simulink model "PID_fin"  (R2023b)
settings: Solver=VariableStepAuto  StartTime=0.0  StopTime=20  RelTol=1e-3
values from neighbouring files (symbols this model uses):
  A = double(A)    [Rotational_inverted_pendulum.m]
  B = double(B)    [Rotational_inverted_pendulum.m]
  C = [1 0 0 0 ... (first row only)    [Rotational_inverted_pendulum.m]
  D = [0 ... (first row only)    [Rotational_inverted_pendulum.m]
  den_phi = cell2mat(G_t2p_uns.Denominator)    [Rotational_inverted_pendulum.m]
  den_theta = cell2mat(G_ol_uns.Denominator(1,1))    [Rotational_inverted_pendulum.m]
  Kd_phi = 60    [Rotational_inverted_pendulum.m]
  Kd_phi_v2 = 0    [Rotational_inverted_pendulum.m]
  Kd_theta = 2    [Rotational_inverted_pendulum.m]
  Kd_theta_v2 = 0.25    [Rotational_inverted_pendulum.m]
  Ki_phi = 50    [Rotational_inverted_pendulum.m]
  Ki_phi_v2 = 7    [Rotational_inverted_pendulum.m]
  Ki_theta = 0    [Rotational_inverted_pendulum.m]
  Ki_theta_v2 = 0    [Rotational_inverted_pendulum.m]
  Kp_phi = 90    [Rotational_inverted_pendulum.m]
  Kp_phi_v2 = 0    [Rotational_inverted_pendulum.m]
  Kp_theta = 5    [Rotational_inverted_pendulum.m]
  Kp_theta_v2 = 0.9    [Rotational_inverted_pendulum.m]
  num_phi = cell2mat(G_t2p_uns.Numerator)    [Rotational_inverted_pendulum.m]
  num_theta = cell2mat(G_ol_uns.Numerator(1,1))    [Rotational_inverted_pendulum.m]
  Va_bar = 0    [Rotational_inverted_pendulum.m]
  x1_bar = double(sol.x1)    [Rotational_inverted_pendulum.m]
  x3_bar = 0    [Rotational_inverted_pendulum.m]
libraries: simulink_extras x5, slpidlib x4
settings Model: Creator=Mark  LastModifiedBy=Mark

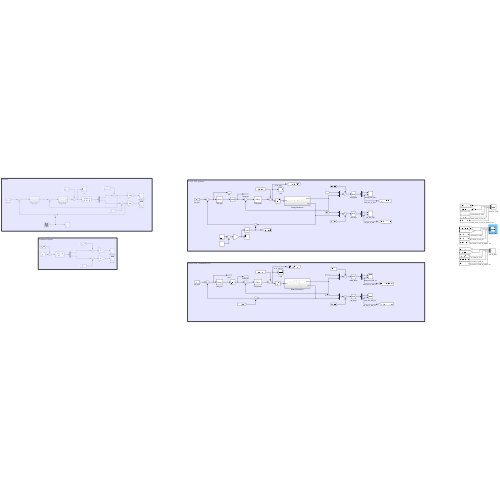
[thumbnail: Simulink's stored preview of the top-level diagram]
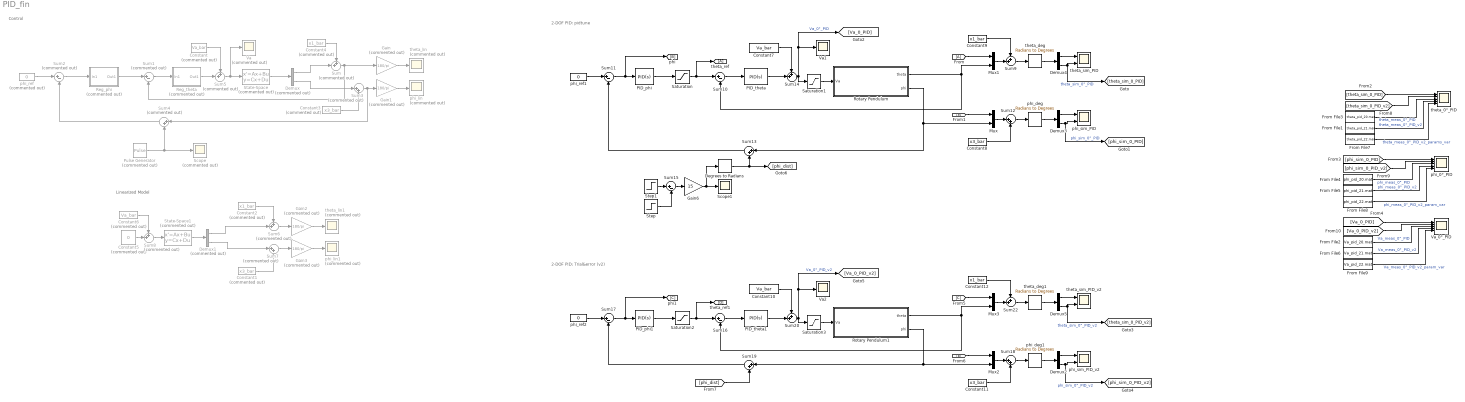
== system PID_fin ==
  note: Control
  note: Linearized Model
  note: 2-DOF PID: pidtune
  note: 2-DOF PID: Trial&error (v2)
  Constant : Constant  Commented=on  Value=Va_bar
  Constant1 : Constant  Commented=on  Value=x3_bar
  Constant10 : Constant  Value=Va_bar
  Constant11 : Constant  Value=x3_bar
  Constant12 : Constant  Value=x1_bar
  Constant2 : Constant  Commented=on  Value=x1_bar
  Constant3 : Constant  Commented=on  Value=x3_bar
  Constant4 : Constant  Commented=on  Value=x1_bar
  Constant5 : Constant  Commented=on  Value=0
  Constant6 : Constant  Commented=on  Value=Va_bar
  Constant7 : Constant  Value=Va_bar
  Constant8 : Constant  Value=x3_bar
  Constant9 : Constant  Value=x1_bar
  Degrees to Radians : simulink_extras/Transformations/Degrees to Radians
  Demux : Demux  Commented=on  Outputs=2
  Demux1 : Demux  Commented=on  Outputs=2
  Demux{2..5} (4 alike) : Demux  Outputs=2
  From : From
  From File1 : FromFile  FileName=theta_pid_21.mat  SampleTime=0
  From File2 : FromFile  FileName=Va_pid_20.mat  SampleTime=0
  From File3 : FromFile  FileName=theta_pid_20.mat  SampleTime=0
  From File4 : FromFile  FileName=phi_pid_20.mat  SampleTime=0
  From File5 : FromFile  FileName=phi_pid_21.mat  SampleTime=0
  From File6 : FromFile  FileName=Va_pid_21.mat  SampleTime=0
  From File7 : FromFile  FileName=theta_pid_22.mat  SampleTime=0
  From File8 : FromFile  FileName=phi_pid_22.mat  SampleTime=0
  From File9 : FromFile  FileName=Va_pid_22.mat  SampleTime=0
  Gain{,1..3} (4 alike) : Gain  Commented=on  Gain=180/pi
  Gain6 : Gain  Gain=15
  Mux{,1..3} (4 alike) : Mux  Inputs=2
  PID_phi : slpidlib/PID Controller  Controller=PID  Form=Parallel  TimeDomain=Continuous-time  UseExternalTs=off  SampleTime=-1  IntegratorMethod=Forward Euler  FilterMethod=Forward Euler  ControllerParametersSource=internal  P=Kp_phi  I=Ki_phi  UseKiTs=off  D=Kd_phi  N=100  UseFilter=on  TunerSelectOption=Transfer Function Based (PID Tuner App)  InitialConditionSource=internal  InitialConditionForIntegrator=0  InitialConditionForFilter=0  DifferentiatorICPrevScaledInput=0  ExternalReset=none  TrackingMode=off  Kt=1  LimitOutput=off  SatLimitsSource=internal  UpperSaturationLimit=90  LowerSaturationLimit=-90  LinearizeAsGain=on  AntiWindupMode=none  Kb=1  LimitIntegrator=off  UpperIntegratorSaturationLimit=inf  LowerIntegratorSaturationLimit=-inf  POutMin=[]  POutMax=[]  IOutMin=[]  IOutMax=[]  DOutMin=[]  DOutMax=[]  NOutMin=[]  NOutMax=[]  SumOutMin=[]  SumOutMax=[]  SaturationOutMin=[]  SaturationOutMax=[]  PParamMin=[]  PParamMax=[]  IParamMin=[]  IParamMax=[]  DParamMin=[]  DParamMax=[]  NParamMin=[]  NParamMax=[]  KbParamMin=[]  KbParamMax=[]  KtParamMin=[]  KtParamMax=[]  KbOutMin=[]  KbOutMax=[]  KtOutMin=[]  KtOutMax=[]  IntegratorOutMin=[]  IntegratorOutMax=[]  FilterOutMin=[]  FilterOutMax=[]  SumI1OutMin=[]  SumI1OutMax=[]  SumI2OutMin=[]  SumI2OutMax=[]  SumI3OutMin=[]  SumI3OutMax=[]  SumI4OutMin=[]  SumI4OutMax=[]  SumDOutMin=[]  SumDOutMax=[]  DifferentiatorOutMin=[]  DifferentiatorOutMax=[]  FilterDiffOutCoefMin=[]  FilterDiffOutCoefMax=[]  ReciprocalOutMin=[]  ReciprocalOutMax=[]  SumDenOutMin=[]  SumDenOutMax=[]  SumNumOutMin=[]  SumNumOutMax=[]  DivideOutMin=[]  DivideOutMax=[]  UdiffTsProdOutMin=[]  UdiffTsProdOutMax=[]  NTsProdOutMin=[]  NTsProdOutMax=[]  UintegralTsProdOutMin=[]  UintegralTsProdOutMax=[]  UngainTsProdOutMin=[]  UngainTsProdOutMax=[]  ClampingZeroOutDataTypeStr=Inherit: Inherit via back propagation  ClampingZeroOutMin=[]  ClampingZeroOutMax=[]  FilterDenConstantOutDataTypeStr=Inherit: Inherit via back propagation  FilterDenConstantOutMin=[]  FilterDenConstantOutMax=[]  PCopyOutDataTypeStr=Inherit: Inherit via back propagation  PCopyOutMin=[]  PCopyOutMax=[]  NCopyOutDataTypeStr=Inherit: Inherit via back propagation  NCopyOutMin=[]  NCopyOutMax=[]  IntegratorContinuousStateAttributes=''  IntegratorStateMustResolveToSignalObject=off  IntegratorRTWStateStorageClass=Auto  FilterContinuousStateAttributes=''  FilterStateMustResolveToSignalObject=off  FilterRTWStateStorageClass=Auto  ParallelPVariant=InternalParameters  IdealPVariant=Disabled  IVariant=InternalParameters  DVariant=InternalParameters  IntegratorVariant=Continuous  SatVariant=Disabled  AWVariant=Passthrough  PCopyVariant=Disabled  TRVariant=Disabled  FdbkBlocksVariant=Forward  IdealPFdbkVariant=Disabled  SatFdbkVariant=Disabled  DerivativeFilterVariant=ContFilter  NVariant=InternalParameters  NCopyVariant=Disabled  FilterICVariant=InternalICsFilter  IntegratorICVariant=InternalICs  ExternalResetVariant=Disabled  TRSumVariant=Passthrough  SumFdbkVariant=Disabled  SumVariant=Sum_PID  TsampFilterVariant=InternalTs  TsampNgainVariant=Passthrough  TsampIntegralVariant=Disabled_SignalSpec  ExternalSaturationOutDataTypeStr=Inherit: Same as second input
  PID_phi1 : slpidlib/PID Controller  Controller=PID  Form=Parallel  TimeDomain=Continuous-time  UseExternalTs=off  SampleTime=-1  IntegratorMethod=Forward Euler  FilterMethod=Forward Euler  ControllerParametersSource=internal  P=Kp_phi_v2  I=Ki_phi_v2  UseKiTs=off  D=Kd_phi_v2  N=100  UseFilter=on  TunerSelectOption=Transfer Function Based (PID Tuner App)  InitialConditionSource=internal  InitialConditionForIntegrator=0  InitialConditionForFilter=0  DifferentiatorICPrevScaledInput=0  ExternalReset=none  TrackingMode=off  Kt=1  LimitOutput=off  SatLimitsSource=internal  UpperSaturationLimit=90  LowerSaturationLimit=-90  LinearizeAsGain=on  AntiWindupMode=none  Kb=1  LimitIntegrator=off  UpperIntegratorSaturationLimit=inf  LowerIntegratorSaturationLimit=-inf  POutMin=[]  POutMax=[]  IOutMin=[]  IOutMax=[]  DOutMin=[]  DOutMax=[]  NOutMin=[]  NOutMax=[]  SumOutMin=[]  SumOutMax=[]  SaturationOutMin=[]  SaturationOutMax=[]  PParamMin=[]  PParamMax=[]  IParamMin=[]  IParamMax=[]  DParamMin=[]  DParamMax=[]  NParamMin=[]  NParamMax=[]  KbParamMin=[]  KbParamMax=[]  KtParamMin=[]  KtParamMax=[]  KbOutMin=[]  KbOutMax=[]  KtOutMin=[]  KtOutMax=[]  IntegratorOutMin=[]  IntegratorOutMax=[]  FilterOutMin=[]  FilterOutMax=[]  SumI1OutMin=[]  SumI1OutMax=[]  SumI2OutMin=[]  SumI2OutMax=[]  SumI3OutMin=[]  SumI3OutMax=[]  SumI4OutMin=[]  SumI4OutMax=[]  SumDOutMin=[]  SumDOutMax=[]  DifferentiatorOutMin=[]  DifferentiatorOutMax=[]  FilterDiffOutCoefMin=[]  FilterDiffOutCoefMax=[]  ReciprocalOutMin=[]  ReciprocalOutMax=[]  SumDenOutMin=[]  SumDenOutMax=[]  SumNumOutMin=[]  SumNumOutMax=[]  DivideOutMin=[]  DivideOutMax=[]  UdiffTsProdOutMin=[]  UdiffTsProdOutMax=[]  NTsProdOutMin=[]  NTsProdOutMax=[]  UintegralTsProdOutMin=[]  UintegralTsProdOutMax=[]  UngainTsProdOutMin=[]  UngainTsProdOutMax=[]  ClampingZeroOutDataTypeStr=Inherit: Inherit via back propagation  ClampingZeroOutMin=[]  ClampingZeroOutMax=[]  FilterDenConstantOutDataTypeStr=Inherit: Inherit via back propagation  FilterDenConstantOutMin=[]  FilterDenConstantOutMax=[]  PCopyOutDataTypeStr=Inherit: Inherit via back propagation  PCopyOutMin=[]  PCopyOutMax=[]  NCopyOutDataTypeStr=Inherit: Inherit via back propagation  NCopyOutMin=[]  NCopyOutMax=[]  IntegratorContinuousStateAttributes=''  IntegratorStateMustResolveToSignalObject=off  IntegratorRTWStateStorageClass=Auto  FilterContinuousStateAttributes=''  FilterStateMustResolveToSignalObject=off  FilterRTWStateStorageClass=Auto  ParallelPVariant=InternalParameters  IdealPVariant=Disabled  IVariant=InternalParameters  DVariant=InternalParameters  IntegratorVariant=Continuous  SatVariant=Disabled  AWVariant=Passthrough  PCopyVariant=Disabled  TRVariant=Disabled  FdbkBlocksVariant=Forward  IdealPFdbkVariant=Disabled  SatFdbkVariant=Disabled  DerivativeFilterVariant=ContFilter  NVariant=InternalParameters  NCopyVariant=Disabled  FilterICVariant=InternalICsFilter  IntegratorICVariant=InternalICs  ExternalResetVariant=Disabled  TRSumVariant=Passthrough  SumFdbkVariant=Disabled  SumVariant=Sum_PID  TsampFilterVariant=InternalTs  TsampNgainVariant=Passthrough  TsampIntegralVariant=Disabled_SignalSpec  ExternalSaturationOutDataTypeStr=Inherit: Same as second input
  PID_theta : slpidlib/PID Controller  Controller=PID  Form=Parallel  TimeDomain=Continuous-time  UseExternalTs=off  SampleTime=-1  IntegratorMethod=Forward Euler  FilterMethod=Forward Euler  ControllerParametersSource=internal  P=Kp_theta  I=Ki_theta  UseKiTs=off  D=Kd_theta  N=100  UseFilter=on  TunerSelectOption=Frequency Response Based  InitialConditionSource=internal  InitialConditionForIntegrator=0  InitialConditionForFilter=0  DifferentiatorICPrevScaledInput=0  ExternalReset=none  TrackingMode=off  Kt=1  LimitOutput=off  SatLimitsSource=internal  UpperSaturationLimit=10  LowerSaturationLimit=-10  LinearizeAsGain=on  AntiWindupMode=back-calculation  Kb=Ki_theta/Kp_theta  LimitIntegrator=off  UpperIntegratorSaturationLimit=inf  LowerIntegratorSaturationLimit=-inf  POutMin=[]  POutMax=[]  IOutMin=[]  IOutMax=[]  DOutMin=[]  DOutMax=[]  NOutMin=[]  NOutMax=[]  SumOutMin=[]  SumOutMax=[]  SaturationOutMin=[]  SaturationOutMax=[]  PParamMin=[]  PParamMax=[]  IParamMin=[]  IParamMax=[]  DParamMin=[]  DParamMax=[]  NParamMin=[]  NParamMax=[]  KbParamMin=[]  KbParamMax=[]  KtParamMin=[]  KtParamMax=[]  KbOutMin=[]  KbOutMax=[]  KtOutMin=[]  KtOutMax=[]  IntegratorOutMin=[]  IntegratorOutMax=[]  FilterOutMin=[]  FilterOutMax=[]  SumI1OutMin=[]  SumI1OutMax=[]  SumI2OutMin=[]  SumI2OutMax=[]  SumI3OutMin=[]  SumI3OutMax=[]  SumI4OutMin=[]  SumI4OutMax=[]  SumDOutMin=[]  SumDOutMax=[]  DifferentiatorOutMin=[]  DifferentiatorOutMax=[]  FilterDiffOutCoefMin=[]  FilterDiffOutCoefMax=[]  ReciprocalOutMin=[]  ReciprocalOutMax=[]  SumDenOutMin=[]  SumDenOutMax=[]  SumNumOutMin=[]  SumNumOutMax=[]  DivideOutMin=[]  DivideOutMax=[]  UdiffTsProdOutMin=[]  UdiffTsProdOutMax=[]  NTsProdOutMin=[]  NTsProdOutMax=[]  UintegralTsProdOutMin=[]  UintegralTsProdOutMax=[]  UngainTsProdOutMin=[]  UngainTsProdOutMax=[]  ClampingZeroOutDataTypeStr=Inherit: Inherit via back propagation  ClampingZeroOutMin=[]  ClampingZeroOutMax=[]  FilterDenConstantOutDataTypeStr=Inherit: Inherit via back propagation  FilterDenConstantOutMin=[]  FilterDenConstantOutMax=[]  PCopyOutDataTypeStr=Inherit: Inherit via back propagation  PCopyOutMin=[]  PCopyOutMax=[]  NCopyOutDataTypeStr=Inherit: Inherit via back propagation  NCopyOutMin=[]  NCopyOutMax=[]  IntegratorContinuousStateAttributes=''  IntegratorStateMustResolveToSignalObject=off  IntegratorRTWStateStorageClass=Auto  FilterContinuousStateAttributes=''  FilterStateMustResolveToSignalObject=off  FilterRTWStateStorageClass=Auto  ParallelPVariant=InternalParameters  IdealPVariant=Disabled  IVariant=InternalParameters  DVariant=InternalParameters  IntegratorVariant=Continuous  SatVariant=Disabled  AWVariant=Passthrough  PCopyVariant=Disabled  TRVariant=Disabled  FdbkBlocksVariant=Forward  IdealPFdbkVariant=Disabled  SatFdbkVariant=Disabled  DerivativeFilterVariant=ContFilter  NVariant=InternalParameters  NCopyVariant=Disabled  FilterICVariant=InternalICsFilter  IntegratorICVariant=InternalICs  ExternalResetVariant=Disabled  TRSumVariant=Passthrough  SumFdbkVariant=Disabled  SumVariant=Sum_PID  TsampFilterVariant=InternalTs  TsampNgainVariant=Passthrough  TsampIntegralVariant=Disabled_SignalSpec  ExternalSaturationOutDataTypeStr=Inherit: Same as second input
  PID_theta1 : slpidlib/PID Controller  Controller=PID  Form=Parallel  TimeDomain=Continuous-time  UseExternalTs=off  SampleTime=-1  IntegratorMethod=Forward Euler  FilterMethod=Forward Euler  ControllerParametersSource=internal  P=Kp_theta_v2  I=Ki_theta_v2  UseKiTs=off  D=Kd_theta_v2  N=100  UseFilter=on  TunerSelectOption=Frequency Response Based  InitialConditionSource=internal  InitialConditionForIntegrator=0  InitialConditionForFilter=0  DifferentiatorICPrevScaledInput=0  ExternalReset=none  TrackingMode=off  Kt=1  LimitOutput=off  SatLimitsSource=internal  UpperSaturationLimit=10  LowerSaturationLimit=-10  LinearizeAsGain=on  AntiWindupMode=back-calculation  Kb=Ki_theta/Kp_theta  LimitIntegrator=off  UpperIntegratorSaturationLimit=inf  LowerIntegratorSaturationLimit=-inf  POutMin=[]  POutMax=[]  IOutMin=[]  IOutMax=[]  DOutMin=[]  DOutMax=[]  NOutMin=[]  NOutMax=[]  SumOutMin=[]  SumOutMax=[]  SaturationOutMin=[]  SaturationOutMax=[]  PParamMin=[]  PParamMax=[]  IParamMin=[]  IParamMax=[]  DParamMin=[]  DParamMax=[]  NParamMin=[]  NParamMax=[]  KbParamMin=[]  KbParamMax=[]  KtParamMin=[]  KtParamMax=[]  KbOutMin=[]  KbOutMax=[]  KtOutMin=[]  KtOutMax=[]  IntegratorOutMin=[]  IntegratorOutMax=[]  FilterOutMin=[]  FilterOutMax=[]  SumI1OutMin=[]  SumI1OutMax=[]  SumI2OutMin=[]  SumI2OutMax=[]  SumI3OutMin=[]  SumI3OutMax=[]  SumI4OutMin=[]  SumI4OutMax=[]  SumDOutMin=[]  SumDOutMax=[]  DifferentiatorOutMin=[]  DifferentiatorOutMax=[]  FilterDiffOutCoefMin=[]  FilterDiffOutCoefMax=[]  ReciprocalOutMin=[]  ReciprocalOutMax=[]  SumDenOutMin=[]  SumDenOutMax=[]  SumNumOutMin=[]  SumNumOutMax=[]  DivideOutMin=[]  DivideOutMax=[]  UdiffTsProdOutMin=[]  UdiffTsProdOutMax=[]  NTsProdOutMin=[]  NTsProdOutMax=[]  UintegralTsProdOutMin=[]  UintegralTsProdOutMax=[]  UngainTsProdOutMin=[]  UngainTsProdOutMax=[]  ClampingZeroOutDataTypeStr=Inherit: Inherit via back propagation  ClampingZeroOutMin=[]  ClampingZeroOutMax=[]  FilterDenConstantOutDataTypeStr=Inherit: Inherit via back propagation  FilterDenConstantOutMin=[]  FilterDenConstantOutMax=[]  PCopyOutDataTypeStr=Inherit: Inherit via back propagation  PCopyOutMin=[]  PCopyOutMax=[]  NCopyOutDataTypeStr=Inherit: Inherit via back propagation  NCopyOutMin=[]  NCopyOutMax=[]  IntegratorContinuousStateAttributes=''  IntegratorStateMustResolveToSignalObject=off  IntegratorRTWStateStorageClass=Auto  FilterContinuousStateAttributes=''  FilterStateMustResolveToSignalObject=off  FilterRTWStateStorageClass=Auto  ParallelPVariant=InternalParameters  IdealPVariant=Disabled  IVariant=InternalParameters  DVariant=InternalParameters  IntegratorVariant=Continuous  SatVariant=Disabled  AWVariant=Passthrough  PCopyVariant=Disabled  TRVariant=Disabled  FdbkBlocksVariant=Forward  IdealPFdbkVariant=Disabled  SatFdbkVariant=Disabled  DerivativeFilterVariant=ContFilter  NVariant=InternalParameters  NCopyVariant=Disabled  FilterICVariant=InternalICsFilter  IntegratorICVariant=InternalICs  ExternalResetVariant=Disabled  TRSumVariant=Passthrough  SumFdbkVariant=Disabled  SumVariant=Sum_PID  TsampFilterVariant=InternalTs  TsampNgainVariant=Passthrough  TsampIntegralVariant=Disabled_SignalSpec  ExternalSaturationOutDataTypeStr=Inherit: Same as second input
  Pulse Generator : DiscretePulseGenerator  Commented=on  PulseType=Time based  Period=10000  PulseWidth=0.01  PhaseDelay=1
  Reg_phi : Subsystem  Commented=on
  Reg_theta : Subsystem  Commented=on
  Rotary Pendulum : Subsystem
  Rotary Pendulum1 : Subsystem
  Saturation : Saturate  UpperLimit=pi/2  LowerLimit=-pi/2
  Saturation1 : Saturate  UpperLimit=10  LowerLimit=-10
  Saturation2 : Saturate  UpperLimit=pi/2  LowerLimit=-pi/2
  Saturation3 : Saturate  UpperLimit=10  LowerLimit=-10
  Scope : Scope  Commented=on
  Scope1 : Scope
  State-Space : StateSpace  Commented=on  A=A  B=B  C=C  D=D  InitialCondition=[0 0 0 0]  ParameterTunability=Optimized
  State-Space1 : StateSpace  Commented=on  A=A  B=B  C=C  D=D  InitialCondition=[0 0 pi/2 0]  ParameterTunability=Optimized
  Step : Step  Time=5.05  SampleTime=0
  Step1 : Step  Time=5  SampleTime=0
  Sum{,5..6,8} (4 alike) : Sum  Commented=on  Inputs=++|
  Sum1 : Sum  Commented=on  Inputs=|+-
  Sum{10..11,15..17} (5 alike) : Sum  Inputs=|+-
  Sum{12..13,18..19} (4 alike) : Sum  Inputs=|++
  Sum{9,14,20,22} (4 alike) : Sum  Inputs=++|
  Sum2 : Sum  Commented=on  Inputs=|+-
  Sum3 : Sum  Commented=on  Inputs=|++
  Sum4 : Sum  Commented=on  Inputs=|++
  Sum7 : Sum  Commented=on  Inputs=|++
  Va : Scope  Commented=on
  Va1 : Scope
  Va2 : Scope
  Va_0°_PID : Scope  NumInputPorts=5
  phi_0°_PID : Scope  NumInputPorts=5
  phi_deg : simulink_extras/Transformations/Radians to Degrees
  phi_deg1 : simulink_extras/Transformations/Radians to Degrees
  phi_lin : Scope  Commented=on
  phi_lin1 : Scope  Commented=on
  phi_ref : Constant  Commented=on  Value=0
  phi_ref1 : Constant  Value=0
  phi_ref2 : Constant  Value=0
  phi_sim_PID : Scope  NumInputPorts=2
  phi_sim_PID_v2 : Scope  NumInputPorts=2
  theta_0°_PID : Scope  NumInputPorts=5
  theta_deg : simulink_extras/Transformations/Radians to Degrees
  theta_deg1 : simulink_extras/Transformations/Radians to Degrees
  theta_lin : Scope  Commented=on
  theta_lin1 : Scope  Commented=on
  theta_ref : Goto
  theta_sim_PID : Scope  NumInputPorts=2
  theta_sim_PID_v2 : Scope  NumInputPorts=2
  wires:
  phi_ref/1 -> Sum2/1
  Reg_phi/1(Out1) -> Sum1/1
  Sum2/1 -> Reg_phi/1(In1)
  State-Space/1 -> Demux/1
  Gain/1 -> theta_lin/1
  Gain1/1 -> phi_lin/1
  Sum/1 -> Gain/1, Sum1/2
  Sum3/1 -> Sum4/1, Gain1/1
  Constant3/1 -> Sum3/2
  Constant4/1 -> Sum/1
  Demux/1 -> Sum/2
  Demux/2 -> Sum3/1
  Sum5/1 -> Va/1, State-Space/1
  Sum1/1 -> Reg_theta/1(In1)
  Sum4/1 -> Sum2/2
  Pulse Generator/1 -> Scope/1, Sum4/2
  Reg_theta/1(Out1) -> Sum5/2
  Constant/1 -> Sum5/1
  Demux1/2 -> Sum7/1
  Sum7/1 -> Gain3/1
  Gain3/1 -> phi_lin1/1
  State-Space1/1 -> Demux1/1
  Demux1/1 -> Sum6/2
  Constant2/1 -> Sum6/1
  Gain2/1 -> theta_lin1/1
  Constant1/1 -> Sum7/2
  Sum6/1 -> Gain2/1
  Constant5/1 -> Sum8/2
  Sum8/1 -> State-Space1/1
  Constant6/1 -> Sum8/1
  phi_ref1/1 -> Sum11/1
  Sum13/1 -> Sum11/2
  Sum10/1 -> PID_theta/1
  Constant9/1 -> Sum9/1
  Sum15/1 -> Gain6/1
  Sum11/1 -> [B], PID_phi/1
  Constant8/1 -> Sum12/2
  Constant7/1 -> Sum14/1
  Gain6/1 -> Scope1/1, Degrees to Radians/1
  From/1 -> Mux1/1
  [B] -> Mux/1
  PID_theta/1 -> Sum14/2
  Sum12/1 -> phi_deg/1
  Sum14/1 -> Saturation1/1, [Va_0_PID], Va1/1  "Va_0°_PID"
  PID_phi/1 -> Saturation/1
  phi_deg/1 -> Demux3/1
  Degrees to Radians/1 -> [phi_dist], Sum13/2
  Mux/1 -> Sum12/1
  Demux3/1 -> phi_sim_PID/1
  Demux3/2 -> [phi_sim_0_PID], phi_sim_PID/2  "phi_sim_0°_PID"
  Mux1/1 -> Sum9/2
  theta_deg/1 -> Demux4/1
  Demux4/1 -> theta_sim_PID/1
  Demux4/2 -> theta_sim_PID/2, [theta_sim_0_PID]  "theta_sim_0°_PID"
  Sum9/1 -> theta_deg/1
  Rotary Pendulum/1(theta) -> Mux1/2, Sum10/2
  Rotary Pendulum/2(phi) -> Sum13/1, Mux/2
  Step/1 -> Sum15/2
  Step1/1 -> Sum15/1
  Saturation/1 -> theta_ref/1, Sum10/1
  Saturation1/1 -> Rotary Pendulum/1(Va)
  [theta_sim_0_PID] -> theta_0°_PID/1
  From File3/1 -> theta_0°_PID/3  "theta_meas_0°_PID"
  [phi_sim_0_PID] -> phi_0°_PID/1
  From File4/1 -> phi_0°_PID/3  "phi_meas_0°_PID"
  [Va_0_PID] -> Va_0°_PID/1
  From File2/1 -> Va_0°_PID/3  "Va_meas_0°_PID"
  Mux2/1 -> Sum18/1
  Sum17/1 -> [C], PID_phi1/1
  theta_deg1/1 -> Demux5/1
  Demux5/1 -> theta_sim_PID_v2/1
  Rotary Pendulum1/2(phi) -> Sum19/1, Mux2/2
  Sum22/1 -> theta_deg1/1
  Demux2/2 -> [phi_sim_0_PID_v2], phi_sim_PID_v2/2  "phi_sim_0°_PID_v2"
  Saturation3/1 -> Rotary Pendulum1/1(Va)
  Mux3/1 -> Sum22/2
  Saturation2/1 -> [D], Sum16/1
  Demux2/1 -> phi_sim_PID_v2/1
  phi_deg1/1 -> Demux2/1
  Sum18/1 -> phi_deg1/1
  [B] -> Mux2/1
  PID_theta1/1 -> Sum20/2
  Rotary Pendulum1/1(theta) -> Mux3/2, Sum16/2
  Sum16/1 -> PID_theta1/1
  Demux5/2 -> theta_sim_PID_v2/2, [theta_sim_0_PID_v2]  "theta_sim_0°_PID_v2"
  Sum20/1 -> Saturation3/1, [Va_0_PID_v2], Va2/1  "Va_0°_PID_v2"
  Constant12/1 -> Sum22/1
  Constant10/1 -> Sum20/1
  phi_ref2/1 -> Sum17/1
  Sum19/1 -> Sum17/2
  [C] -> Mux3/1
  Constant11/1 -> Sum18/2
  PID_phi1/1 -> Saturation2/1
  [phi_dist] -> Sum19/2
  [theta_sim_0_PID_v2] -> theta_0°_PID/2
  [phi_sim_0_PID_v2] -> phi_0°_PID/2
  [Va_0_PID_v2] -> Va_0°_PID/2
  From File1/1 -> theta_0°_PID/4  "theta_meas_0°_PID_v2"
  From File5/1 -> phi_0°_PID/4  "phi_meas_0°_PID_v2"
  From File6/1 -> Va_0°_PID/4  "Va_meas_0°_PID_v2"
  From File7/1 -> theta_0°_PID/5  "theta_meas_0°_PID_v2_params_var"
  From File8/1 -> phi_0°_PID/5  "phi_meas_0°_PID_v2_param_var"
  From File9/1 -> Va_0°_PID/5  "Va_meas_0°_PID_v2_param_var"

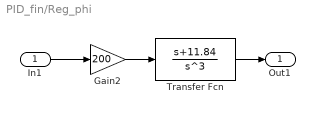
== system PID_fin/Reg_phi ==
  In1 : Inport
  Gain2 : Gain  Gain=200
  Transfer Fcn : TransferFcn  Numerator=[1 11.84]  Denominator=[1 0 0 0]
  Out1 : Outport
  wires:
  Gain2/1 -> Transfer Fcn/1
  Transfer Fcn/1 -> Out1/1
  In1/1 -> Gain2/1

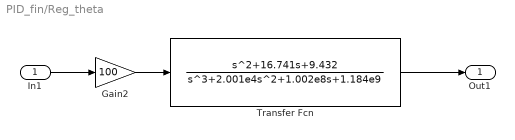
== system PID_fin/Reg_theta ==
  In1 : Inport
  Gain2 : Gain  Gain=100
  Transfer Fcn : TransferFcn  Numerator=[1 16.741 9.432]  Denominator=[1 2.001e4 1.002e8 1.184e9]
  Out1 : Outport
  wires:
  Gain2/1 -> Transfer Fcn/1
  Transfer Fcn/1 -> Out1/1
  In1/1 -> Gain2/1

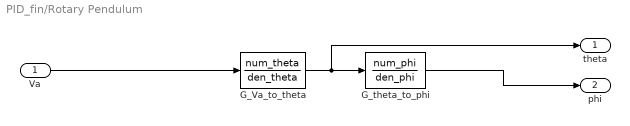
== system PID_fin/Rotary Pendulum ==
  Va : Inport
  G_Va_to_theta : TransferFcn  Numerator=num_theta  Denominator=den_theta
  G_theta_to_phi : TransferFcn  Numerator=num_phi  Denominator=den_phi
  theta : Outport
  phi : Outport  Port=2
  wires:
  G_theta_to_phi/1 -> phi/1
  G_Va_to_theta/1 -> theta/1, G_theta_to_phi/1
  Va/1 -> G_Va_to_theta/1

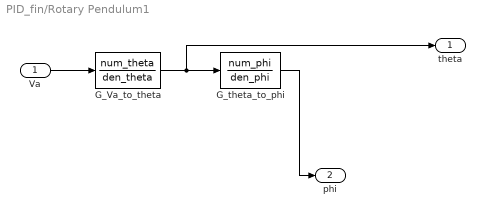
== system PID_fin/Rotary Pendulum1 ==
  Va : Inport
  G_Va_to_theta : TransferFcn  Numerator=num_theta  Denominator=den_theta
  G_theta_to_phi : TransferFcn  Numerator=num_phi  Denominator=den_phi
  theta : Outport
  phi : Outport  Port=2
  wires:
  G_theta_to_phi/1 -> phi/1
  G_Va_to_theta/1 -> theta/1, G_theta_to_phi/1
  Va/1 -> G_Va_to_theta/1
